simulink model "sensores_no_ideales_desagregado"  (R2023b)
settings: Solver=VariableStepAuto  StartTime=0.0  StopTime=10.0  RelTol=1e-3
undefined symbols (not defined in the file or in its folder): gain_i_1, gain_i_2, gain_pos_1, gain_pos_2, gain_T, X0_ia, X0_ib, X0_ic, X0_pos, X0_T
settings Model: Creator=Pc  LastModifiedBy=Gabriel

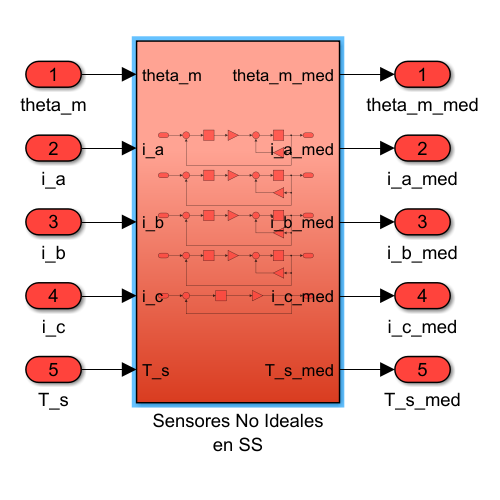
[thumbnail: Simulink's stored preview of the top-level diagram]
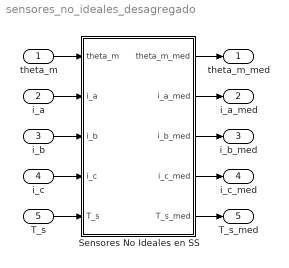
== system sensores_no_ideales_desagregado ==
  theta_m : Inport
  i_a : Inport  Port=2
  i_b : Inport  Port=3
  i_c : Inport  Port=4
  T_s : Inport  Port=5
  Sensores No Ideales en SS : Subsystem
  theta_m_med : Outport
  i_a_med : Outport  Port=2
  i_b_med : Outport  Port=3
  i_c_med : Outport  Port=4
  T_s_med : Outport  Port=5
  wires:
  theta_m/1 -> Sensores No Ideales en SS/1(theta_m)
  i_a/1 -> Sensores No Ideales en SS/2(i_a)
  i_b/1 -> Sensores No Ideales en SS/3(i_b)
  i_c/1 -> Sensores No Ideales en SS/4(i_c)
  T_s/1 -> Sensores No Ideales en SS/5(T_s)
  Sensores No Ideales en SS/1(theta_m_med) -> theta_m_med/1
  Sensores No Ideales en SS/2(i_a_med) -> i_a_med/1
  Sensores No Ideales en SS/3(i_b_med) -> i_b_med/1
  Sensores No Ideales en SS/4(i_c_med) -> i_c_med/1
  Sensores No Ideales en SS/5(T_s_med) -> T_s_med/1

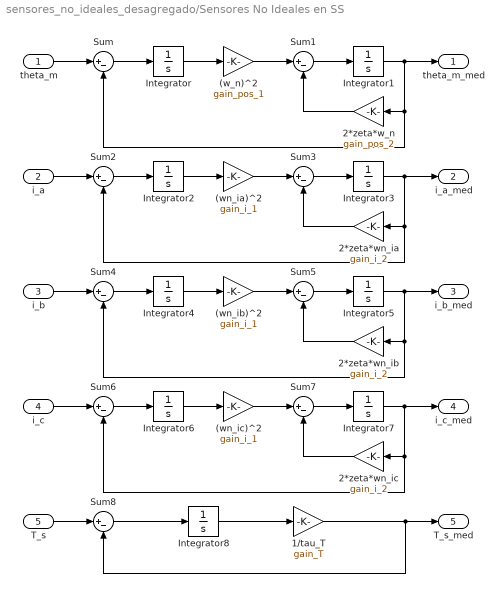
== system sensores_no_ideales_desagregado/Sensores No Ideales en SS ==
  theta_m : Inport
  i_a : Inport  Port=2
  i_b : Inport  Port=3
  i_c : Inport  Port=4
  T_s : Inport  Port=5
  (w_n)^2 : Gain  Gain=gain_pos_1
  (wn_ia)^2 : Gain  Gain=gain_i_1
  (wn_ib)^2 : Gain  Gain=gain_i_1
  (wn_ic)^2 : Gain  Gain=gain_i_1
  1/tau_T : Gain  Gain=gain_T
  2*zeta*w_n : Gain  Gain=gain_pos_2
  2*zeta*wn_ia : Gain  Gain=gain_i_2
  2*zeta*wn_ib : Gain  Gain=gain_i_2
  2*zeta*wn_ic : Gain  Gain=gain_i_2
  Integrator : Integrator  InitialCondition=X0_pos(1)
  Integrator1 : Integrator  InitialCondition=X0_pos(2)
  Integrator2 : Integrator  InitialCondition=X0_ia(1)
  Integrator3 : Integrator  InitialCondition=X0_ia(2)
  Integrator4 : Integrator  InitialCondition=X0_ib(1)
  Integrator5 : Integrator  InitialCondition=X0_ib(2)
  Integrator6 : Integrator  InitialCondition=X0_ic(1)
  Integrator7 : Integrator  InitialCondition=X0_ic(2)
  Integrator8 : Integrator  InitialCondition=X0_T
  Sum{,1..8} (9 alike) : Sum  Inputs=|+-
  theta_m_med : Outport
  i_a_med : Outport  Port=2
  i_b_med : Outport  Port=3
  i_c_med : Outport  Port=4
  T_s_med : Outport  Port=5
  wires:
  i_a/1 -> Sum2/1
  theta_m/1 -> Sum/1
  Sum/1 -> Integrator/1
  Integrator/1 -> (w_n)^2/1
  (w_n)^2/1 -> Sum1/1
  2*zeta*w_n/1 -> Sum1/2
  Sum1/1 -> Integrator1/1
  Integrator1/1 -> theta_m_med/1, Sum/2, 2*zeta*w_n/1
  Integrator3/1 -> i_a_med/1, 2*zeta*wn_ia/1, Sum2/2
  Sum3/1 -> Integrator3/1
  2*zeta*wn_ia/1 -> Sum3/2
  (wn_ia)^2/1 -> Sum3/1
  Integrator2/1 -> (wn_ia)^2/1
  Sum2/1 -> Integrator2/1
  Sum4/1 -> Integrator4/1
  Integrator4/1 -> (wn_ib)^2/1
  (wn_ib)^2/1 -> Sum5/1
  2*zeta*wn_ib/1 -> Sum5/2
  Sum5/1 -> Integrator5/1
  Integrator5/1 -> i_b_med/1, Sum4/2, 2*zeta*wn_ib/1
  i_b/1 -> Sum4/1
  Integrator7/1 -> i_c_med/1, 2*zeta*wn_ic/1, Sum6/2
  Sum7/1 -> Integrator7/1
  2*zeta*wn_ic/1 -> Sum7/2
  (wn_ic)^2/1 -> Sum7/1
  Integrator6/1 -> (wn_ic)^2/1
  Sum6/1 -> Integrator6/1
  i_c/1 -> Sum6/1
  Sum8/1 -> Integrator8/1
  Integrator8/1 -> 1/tau_T/1
  T_s/1 -> Sum8/1
  1/tau_T/1 -> Sum8/2, T_s_med/1
